simulink model "Cascade_realization"  (R2020a)
settings: Solver=VariableStepAuto  StartTime=0.0  StopTime=10.0  RelTol=1e-3
settings Model: Creator=Shivam  LastModifiedBy=Shivam

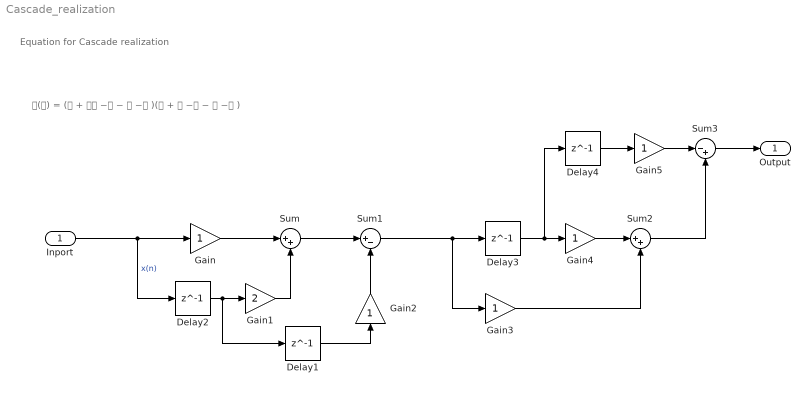
== system Cascade_realization ==
  note: 𝐇(𝐳) = (𝟏 + 𝟐𝐳 −𝟏 − 𝐳 −𝟐 )(𝟏 + 𝐳 −𝟏 − 𝐳 −𝟐 )
  note: Equation for Cascade realization
  Inport : Inport
  Delay{1..4} (4 alike) : Delay  DelayLength=1
  Gain{,2..5} (5 alike) : Gain
  Gain1 : Gain  Gain=2
  Sum : Sum  Inputs=|++
  Sum1 : Sum  Inputs=|+-
  Sum2 : Sum  Inputs=|++
  Sum3 : Sum  Inputs=|-+
  Output : Outport
  wires:
  Inport/1 -> Gain/1, Delay2/1  "x(n)"
  Gain/1 -> Sum/1
  Delay2/1 -> Delay1/1, Gain1/1
  Gain1/1 -> Sum/2
  Sum/1 -> Sum1/1
  Delay1/1 -> Gain2/1
  Gain2/1 -> Sum1/2
  Sum1/1 -> Gain3/1, Delay3/1
  Delay3/1 -> Delay4/1, Gain4/1
  Gain4/1 -> Sum2/1
  Gain3/1 -> Sum2/2
  Delay4/1 -> Gain5/1
  Gain5/1 -> Sum3/1
  Sum2/1 -> Sum3/2
  Sum3/1 -> Output/1
